simulink model "DSimulator_robot3GDL"  (R2021b)
settings: Solver=ode1  StartTime=0  StopTime=500  FixedStep=0.0004  RelTol=1e-3  EnableMultiTasking=on
undefined symbols (not defined in the file or in its folder): Dinamic_ur10_3DOF, disp_q, SimpleRobotPlotROS, Tau, TrajGen
libraries: simulink x3
settings Model: Creator=E. Dean  LastModifiedBy=redball
settings SolverCC: AlgebraicLoopSolver=TrustRegion
settings DataIOCC: LimitDataPoints=on  SaveFormat=Array  SignalLoggingSaveFormat=ModelDataLogs  ReturnWorkspaceOutputs=off
settings OptimizationCC: ExpressionDepthLimit=2147483647  LifeSpan=inf
settings DebuggingCC: UnderspecifiedInitializationDetection=Classic  MergeDetectMultiDrivingBlocksExec=none  SolverPrmCheckMsg=warning  FcnCallInpInsideContextMsg=warning  AllowSymbolicDim=off  StateNameClashWarn=warning  SFUnexpectedBacktrackingDiag=warning  SFNoUnconditionalDefaultTransitionDiag=warning  SFExecutionAtInitializationDiag=none  SFMachineParentedDataDiag=warning  ArithmeticOperatorsInVariantConditions=warning
settings HardwareCC: ProdBitPerPointer=32  ProdBitPerSizeT=32  ProdBitPerPtrDiffT=32  ProdLargestAtomicFloat=None  ProdIntDivRoundTo=Undefined  ProdEndianess=Unspecified  ProdWordSize=32  ProdHWDeviceType=32-bit Generic
settings ModelReferenceCC: PropagateSignalLabelsOutOfModel=off
settings SFSimCC: SimUseLocalCustomCode=off  CustomCodeUndefinedFunction=UseInterfaceOnly
settings RTWCC: RTWUseLocalCustomCode=off
settings CodeAppCC: StateflowObjectComments=on
settings GRTTargetCC: TargetLangStandard=C89/C90 (ANSI)  CombineOutputUpdateFcns=off  GRTInterface=on
settings ConfigComp: CovMetricSettings=dw  CovSaveCumulativeToWorkspaceVar=on  CovSaveSingleToWorkspaceVar=on  CovExternalEMLEnable=off  CovSFcnEnable=off

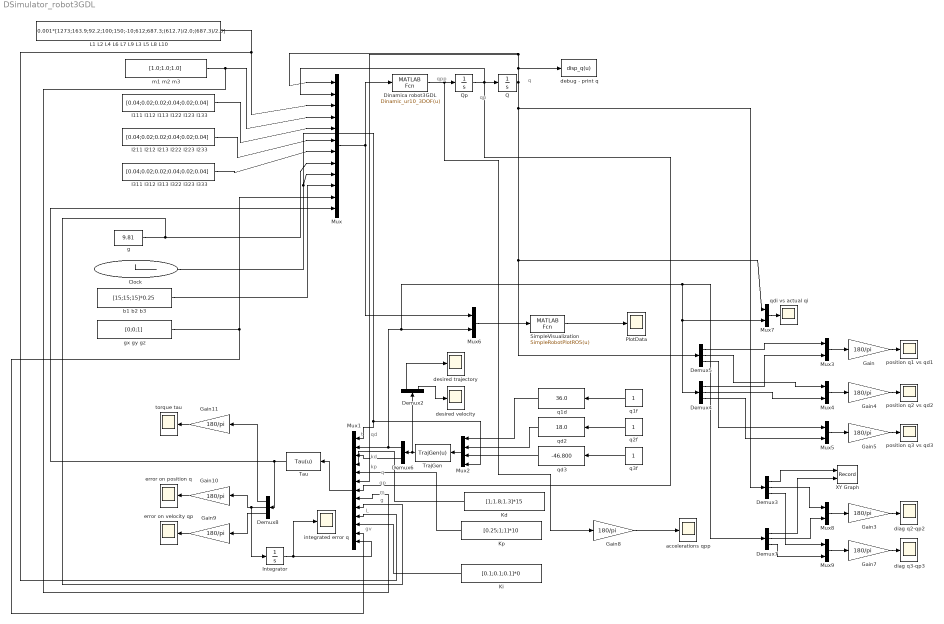
== system DSimulator_robot3GDL ==
  note: gv
  note: qd
  note: q
  note: qp
  note: qpp
  note: t
  note: L
  note: g
  note: m
  note: kp
  note: kd
  note: qp
  note: q
  Clock : Clock
  Demux2 : Demux  Outputs=2
  Demux{3..5,7..8} (5 alike) : Demux  Outputs=3
  Demux6 : Demux  Outputs=2
  Dinamica robot3GDL : MATLABFcn  MATLABFcn=Dinamic_ur10_3DOF(u)  OutputDimensions=6
  Gain{,3..5,7..11} (9 alike) : Gain  Gain=180/pi
  I111 I112 I113 I122 I123 I133 : Constant  Value=[0.04;0.02;0.02;0.04;0.02;0.04]
  I211 I212 I213 I222 I223 I233 : Constant  Value=[0.04;0.02;0.02;0.04;0.02;0.04]
  I311 I312 I313 I322 I323 I333 : Constant  Value=[0.04;0.02;0.02;0.04;0.02;0.04]
  Integrator : Integrator
  "Kd " : Constant  Value=[1;1.8;1.3]*15
  Ki : Constant  Value=[0.1;0.1;0.1]*0
  Kp : Constant  Value=[0.25;1;1]*10
  "L1 L2 L4 L6 L7 L9 L3 L5 L8 L10 " : Constant  Value=0.001*[1273;163.9;92.2;100;150;-10;612;687.3;(612.7)/2.0;(687.3)/2.0]
  Mux : Mux  Inputs=12
  Mux1 : Mux  Inputs=13
  Mux2 : Mux
  Mux{3..9} (7 alike) : Mux  Inputs=2
  PlotData : Scope
  Q : Integrator  InitialCondition=[0;0;0;0;0;0]
  Qp : Integrator  InitialCondition=[0;0;0;0;0;0]
  SimpleVisualization : MATLABFcn  MATLABFcn=SimpleRobotPlotROS(u)  OutputDimensions=3
  "Tau " : MATLABFcn  MATLABFcn=Tau(u)  OutputDimensions=9
  TrajGen : MATLABFcn  MATLABFcn=TrajGen(u)  OutputDimensions=6
  XY Graph : Record  FileSettingsInternal="{\"entries\":[{\"content\":{\"excelSettings\":{\"content\":{},\"type\":\"Streamout.ExcelSettings\"}},\"type\":\"Streamout.FileSettingStorage\",\"uuid\":\"7e91849d-0305-4a47-b699-66653e6078aa\"}],\"packageUris\":[\"http://schema.mathworks.com/mf0/streamout_blocks/R2020a\"],\"version\":\"1.0\"}"  Layout=[1 1]  SignalsInternal="{\"entries\":[{\"content\":{\"signals\":[{\"content\":{\"blockPath\":[\"DSimulator_robot3GDL/XY Graph\"],\"channel\":[],\"dimensions\":[2],\"domain\":\"DSimulator_robot3GDL/XY Graph\",\"hasChildren\":true,\"lineColor\":\"#ff6929\",\"plots\":[],\"port\":1,\"sid\":[\"\"],\"signalID\":343,\"signalName\":\"Demux3:1\"},\"type\":\"RecordBlkView.Signal\",\"uuid\":\"ce1ae430-1b99-43bc-b0e8-25b652dc7590\"},{\"content\":{\"blockPath\":[\"DSimulator_robot3GDL/XY Graph\"],\"channel\":[1],\"dimensions\":[2],\"domain\":\"DSimulator_robot3GDL/XY Graph\",\"lineColor\":\"#ff13a6\",\"parentID\":343,\"plots\":[],\"port\":1,\"sid\":[\"\"],\"signalID\":344,\"signalName\":\"Demux3:1\"},\"type\":\"RecordBlkView.Signal\",\"uuid\":\"c00e818e-be77-4ca0-b0de-e65e8b7d85cf\"},{\"content\":{\"blockPath\":[\"DSimulator_robot3GDL/XY Graph\"],\"channel\":[],\"dimensions\":[1],\"domain\":\"DSimulator_robot3GDL/XY Graph\",\"lineColor\":\"#139fff\",\"plots\":[1],\"port\":2,\"sid\":[\"\"],\"signalID\":348,\"signalName\":\"Demux7:1\"},\"type\":\"RecordBlkView.Signal\",\"uuid\":\"be9bb1d7-8b14-4f48-9669-03951ca7a638\"},{\"content\":{\"blockPath\":[\"DSimulator_robot3GDL/XY Graph\"],\"channel\":[2],\"dimensions\":[2],\"domain\":\"DSimulator_robot3GDL/XY Graph\",\"lineColor\":\"#edb120\",\"parentID\":343,\"plots\":[],\"port\":1,\"sid\":[\"\"],\"signalID\":352,\"signalName\":\"Demux3:1\"},\"type\":\"RecordBlkView.Signal\",\"uuid\":\"c75284fc-b204-4ce1-94a6-54a3b7531d4d\"}]},\"type\":\"RecordBlkView.InputSignals\",\"uuid\":\"e807ccfc-4967-4d79-8a18-ed7df802d3a5\"}],\"packageUris\":[\"http://schema.mathworks.com/mf0/streamout_blocks/R2020a\"],\"version\":\"1.0\"}"  VisualizationBindings="{\"xyplotplugin\":{\"info\":[{\"series\":[{\"bindingParametersList\":[{\"parameter\":\"Y-Axis\",\"signalID\":348,\"signalName\":\"Demux7:1\"}],\"seriesID\":17835}],\"subplotID\":1}]}}"  CompatibilityTag=XY
  accelerations qpp : Scope
  "b1 b2 b3 " : Constant  Value=[15;15;15]*0.25
  debug - print q : MATLABFcn  MATLABFcn=disp_q(u)  OutputDimensions=0
  desired trajectory : Scope
  desired velocity : Scope
  diag q2-qp2 : Scope
  diag q3-qp3 : Scope
  error on position q : Scope
  error on velocity qp : Scope
  g : Constant  Value=9.81
  gx gy gz : Constant  Value=[0;0;1]
  integrated error q : Scope
  "m1 m2 m3 " : Constant  Value=[1.0;1.0;1.0]
  position q1 vs qd1 : Scope
  position q2 vs qd2 : Scope
  position q3 vs qd3 : Scope
  q1d : simulink/Math Operations/Slider Gain  gain=36.0  low=-180  high=180
  q1f : Constant
  q2f : Constant
  q3f : Constant
  qd2 : simulink/Math Operations/Slider Gain  gain=18.0  low=-180  high=180
  qd3 : simulink/Math Operations/Slider Gain  gain=-46.800  low=-180  high=180
  qdi vs actual qi : Scope
  torque tau : Scope
  wires:
  Dinamica robot3GDL/1 -> Gain8/1, Qp/1
  Gain/1 -> position q1 vs qd1/1
  I111 I112 I113 I122 I123 I133/1 -> Mux/5
  I211 I212 I213 I222 I223 I233/1 -> Mux/6
  I311 I312 I313 I322 I323 I333/1 -> Mux/7
  "b1 b2 b3 "/1 -> Mux/10
  SimpleVisualization/1 -> PlotData/1
  Mux/1 -> Mux6/1, Dinamica robot3GDL/1
  Mux1/1 -> "Tau "/1
  q1f/1 -> q1d/1
  q2f/1 -> qd2/1
  q3f/1 -> qd3/1
  q1d/1 -> Mux2/1
  qd2/1 -> Mux2/2
  "Kd "/1 -> Mux1/4
  Kp/1 -> Mux1/5
  Q/1 -> Demux5/1, Mux7/1, Demux3/1, debug - print q/1, Mux/1, Mux1/6
  Qp/1 -> Q/1, Mux1/7, Mux/2
  "m1 m2 m3 "/1 -> Mux1/8, Mux/4
  g/1 -> Mux1/9, Mux/8
  "L1 L2 L4 L6 L7 L9 L3 L5 L8 L10 "/1 -> Mux1/10, Mux/3
  Clock/1 -> Mux2/4, Mux1/1, Mux/9
  Ki/1 -> Mux1/11
  Demux4/1 -> Mux3/2
  Mux3/1 -> Gain/1
  Gain4/1 -> position q2 vs qd2/1
  Mux4/1 -> Gain4/1
  Gain5/1 -> position q3 vs qd3/1
  Mux5/1 -> Gain5/1
  Demux5/1 -> Mux3/1
  Demux5/2 -> Mux4/1
  Mux6/1 -> SimpleVisualization/1
  "Tau "/1 -> Demux8/1, Mux/12
  gx gy gz/1 -> Mux1/12, Mux/11
  Demux5/3 -> Mux5/1
  Demux4/2 -> Mux4/2
  Demux4/3 -> Mux5/2
  TrajGen/1 -> Demux2/1, Demux6/1
  Demux6/1 -> Mux1/2, Mux7/2, Demux4/1, Demux7/1, Mux6/2
  Demux6/2 -> Mux1/3
  Demux2/1 -> desired trajectory/1
  Gain3/1 -> diag q2-qp2/1
  Gain7/1 -> diag q3-qp3/1
  Mux8/1 -> Gain3/1
  Mux9/1 -> Gain7/1
  Demux3/1 -> XY Graph/1
  Demux7/1 -> XY Graph/2
  Demux3/2 -> Mux8/1
  Demux7/2 -> Mux8/2
  Demux3/3 -> Mux9/1
  Demux7/3 -> Mux9/2
  Gain10/1 -> error on position q/1
  Gain9/1 -> error on velocity qp/1
  Demux8/2 -> Integrator/1, Gain10/1
  Demux8/3 -> Gain9/1
  Gain8/1 -> accelerations qpp/1
  Demux8/1 -> Gain11/1
  Gain11/1 -> torque tau/1
  Integrator/1 -> Mux1/13, integrated error q/1
  Demux2/2 -> desired velocity/1
  Mux2/1 -> TrajGen/1
  qd3/1 -> Mux2/3
  Mux7/1 -> qdi vs actual qi/1
